simulink model "FmTest"  (R2024b)
settings: Solver=VariableStepAuto  StartTime=0.0  StopTime=10.0  RelTol=1e-3
values from neighbouring files (symbols this model uses):
  CanaryCarrierFrequency = 20000.0    [ConfigData.sldd]
  CanaryDataRate = 100.0    [ConfigData.sldd]
  SampleRate = 48000.0    [ConfigData.sldd]
  WalshCodeIndex = 9.0 3.0    [ConfigData.sldd]
undefined symbols (not defined in the file or in its folder): DiscIntNeverNeededParam
libraries: dspfdesign x4, dspsnks4 x2, commseqgen3 x2, eeGeneralControl x1
settings Model: DataDictionary=ConfigData.sldd  SimulationMode=accelerator  Creator=calum  LastModifiedBy=calum

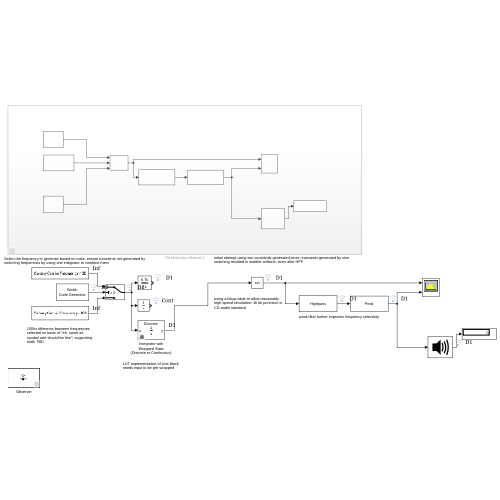
[thumbnail: Simulink's stored preview of the top-level diagram]
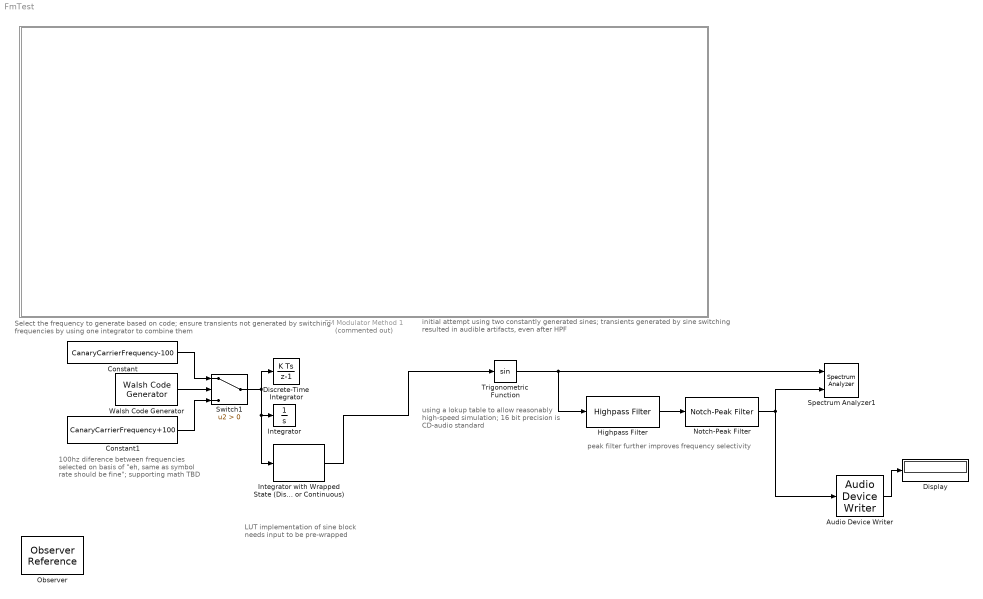
== system FmTest ==
  note: Select the frequency to generate based on code; ensure transients not generated by switching frequencies by using one integrator to combine them
  note: initial attempt using two constantly generated sines; transients generated by sine switching resulted in audible artifacts, even after HPF
  note: LUT implementation of sine block needs input to be pre-wrapped
  note: 100hz diference between frequencies selected on basis of "eh, same as symbol rate should be fine"; supporting math TBD
  note: peak filter further improves frequency selectivity
  note: using a lokup table to allow reasonably high-speed simulation; 16 bit precision is CD-audio standard
  Audio Device Writer : dspsnks4/Audio Device Writer  Driver=ALSA  Device=pipewire  InheritSampleRate=off  SampleRate=SampleRate  BitDepth=32-bit float  BufferSize=4096  NumBuffers=10  DefaultOutputChannelMapping=on  OutputChannelMapping=1:2  OutputNumUnderrunSamples=on  DriverIdx=8  DeviceWarnFlag=''
  Constant : Constant  Value=CanaryCarrierFrequency-100
  Constant1 : Constant  Value=CanaryCarrierFrequency+100
  Discrete-Time Integrator : DiscreteIntegrator  gainval=1  SampleTime=1/SampleRate  ICPrevOutput=DiscIntNeverNeededParam  ICPrevScaledInput=DiscIntNeverNeededParam
  Display : Display
  FM Modulator Method 1 : Subsystem  Commented=on
  Highpass Filter : dspfdesign/Highpass Filter  FilterType=FIR  DesignForMinimumOrder=on  FilterOrder=50  StopbandFrequency=CanaryCarrierFrequency-1000  PassbandFrequency=CanaryCarrierFrequency  StopbandAttenuation=80  PassbandRipple=0.1  SampleRateMode=Specify on dialog  SampleRate=SampleRate  SimulateUsing=Code generation  roundingMode=Floor  coeffsDataTypeStr=fixdt(1,16)
  Integrator : Integrator
  Integrator with Wrapped State (Discrete or Continuous) : eeGeneralControl/Integrator with Wrapped State (Discrete or Continuous)  LabelModeActiveChoice=Discrete  WrappedStateUpperValue=1  WrappedStateLowerValue=0  x0=0  Ts=1/SampleRate
      settings: LibrarySourceBlock=|
      | ee_sl_lib/General Control/Integrator with
      | Wrapped State
      | (Discrete or Continuous)
  Notch-Peak Filter : dspfdesign/Notch-Peak Filter  Specification=Bandwidth and center frequency  BandwidthPort=off  Bandwidth=CanaryDataRate  QualityFactorPort=off  QualityFactor=5  CenterFrequencyPort=off  CenterFrequency=CanaryCarrierFrequency  BandwidthCoefficientPort=off  BandwidthCoefficient=0.72654  CenterFrequencyCoefficientPort=off  CenterFrequencyCoefficient=0  Output=Peak  SampleRateMode=Specify on dialog  SampleRate=SampleRate  SimulateUsing=Code generation
  Observer : ObserverReference  ObserverModelName=FmTest_Observer1
  Spectrum Analyzer1 : SpectrumAnalyzer  NumInputPorts=2  WindowPosition=[1.000000,1.000000,1920.000000,1003.000000,]  Visible=on  ScopeFrameLocation=window  SampleRate=44.1e3  PlotAsTwoSidedSpectrum=off  FrequencyScale=Log  WindowInvariantSamplesPerUpdate=on  StartFrequency=20  StopFrequency=20e3  YLimits=[-176.71181838,42.92763292]  SelectedToolstripTab=spectrumAnalyzerToolstrip.estimationTab
  Switch1 : Switch  Criteria=u2 > Threshold  SaturateOnIntegerOverflow=off  InputSameDT=off
  Trigonometric Function : Trigonometry  ApproximationMethod=Lookup  AngleUnit=revolution  NumberOfDataPoints=(2^16)+1
  Walsh Code Generator : commseqgen3/Walsh Code Generator  Length=16  Index=WalshCodeIndex(2)  SampleTime=1/CanaryDataRate  SamplesPerFrame=1  OutputDataType=double  SimulateUsing=Code generation
  wires:
  Walsh Code Generator/1 -> Switch1/2
  Switch1/1 -> Discrete-Time Integrator/1, Integrator with Wrapped State (Discrete or Continuous)/1, Integrator/1
  Constant/1 -> Switch1/1
  Constant1/1 -> Switch1/3
  Audio Device Writer/1 -> Display/1
  Highpass Filter/1 -> Notch-Peak Filter/1
  Trigonometric Function/1 -> Highpass Filter/1, Spectrum Analyzer1/1
  Notch-Peak Filter/1 -> Audio Device Writer/1, Spectrum Analyzer1/2
  Integrator with Wrapped State (Discrete or Continuous)/1 -> Trigonometric Function/1

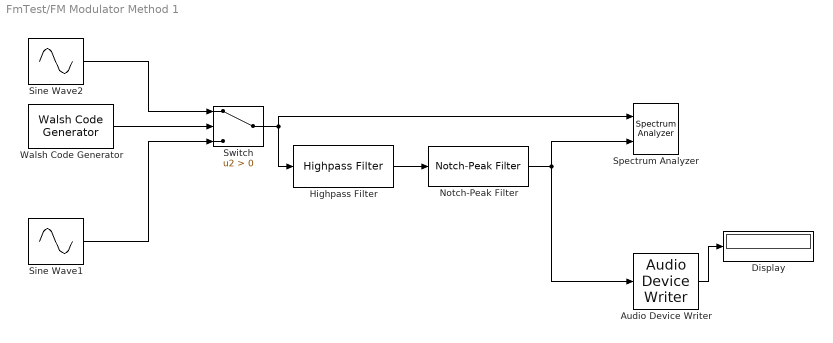
== system FmTest/FM Modulator Method 1 ==
  Audio Device Writer : dspsnks4/Audio Device Writer  Driver=ALSA  Device=pipewire  InheritSampleRate=off  SampleRate=SampleRate  BitDepth=32-bit float  BufferSize=4096  NumBuffers=10  DefaultOutputChannelMapping=on  OutputChannelMapping=1:2  OutputNumUnderrunSamples=on  DriverIdx=8  DeviceWarnFlag=''
  Display : Display
  Highpass Filter : dspfdesign/Highpass Filter  FilterType=FIR  DesignForMinimumOrder=on  FilterOrder=50  StopbandFrequency=CanaryCarrierFrequency-1000  PassbandFrequency=CanaryCarrierFrequency  StopbandAttenuation=80  PassbandRipple=0.1  SampleRateMode=Specify on dialog  SampleRate=SampleRate  SimulateUsing=Code generation  roundingMode=Floor  coeffsDataTypeStr=fixdt(1,16)
  Notch-Peak Filter : dspfdesign/Notch-Peak Filter  Specification=Bandwidth and center frequency  BandwidthPort=off  Bandwidth=CanaryDataRate  QualityFactorPort=off  QualityFactor=5  CenterFrequencyPort=off  CenterFrequency=CanaryCarrierFrequency  BandwidthCoefficientPort=off  BandwidthCoefficient=0.72654  CenterFrequencyCoefficientPort=off  CenterFrequencyCoefficient=0  Output=Peak  SampleRateMode=Specify on dialog  SampleRate=SampleRate  SimulateUsing=Code generation
  Sine Wave1 : Sin  Frequency=(CanaryCarrierFrequency+CanaryDataRate)*2*pi  SampleTime=1/SampleRate
  Sine Wave2 : Sin  Frequency=(CanaryCarrierFrequency-CanaryDataRate)*2*pi  SampleTime=1/SampleRate
  Spectrum Analyzer : SpectrumAnalyzer  NumInputPorts=2  WindowPosition=[1.000000,1.000000,1920.000000,1003.000000,]  ScopeFrameLocation=window  SampleRate=44.1e3  PlotAsTwoSidedSpectrum=off  FrequencyScale=Log  WindowInvariantSamplesPerUpdate=on  StartFrequency=20  StopFrequency=20e3  YLimits=[-118.03026141,36.42915272]  SelectedToolstripTab=spectrumAnalyzerToolstrip.estimationTab
  Switch : Switch  Criteria=u2 > Threshold  SaturateOnIntegerOverflow=off  InputSameDT=off
  Walsh Code Generator : commseqgen3/Walsh Code Generator  Length=16  Index=WalshCodeIndex(2)  SampleTime=1/CanaryDataRate  SamplesPerFrame=1  OutputDataType=double  SimulateUsing=Code generation
  wires:
  Audio Device Writer/1 -> Display/1
  Sine Wave2/1 -> Switch/1
  Walsh Code Generator/1 -> Switch/2
  Notch-Peak Filter/1 -> Audio Device Writer/1, Spectrum Analyzer/2
  Highpass Filter/1 -> Notch-Peak Filter/1
  Switch/1 -> Spectrum Analyzer/1, Highpass Filter/1
  Sine Wave1/1 -> Switch/3
